simulink model "test_on_intes_cross2018_acc"  (R2018b)
settings: Solver=FixedStepAuto  StartTime=0.0  StopTime=10.0  FixedStep=0.001  RelTol=1e-3
libraries: simulink x1
settings Model: Creator=lenovo  LastModifiedBy=lenovo

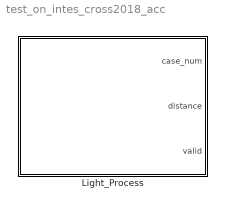
== system test_on_intes_cross2018_acc ==
  Light_Process : Subsystem

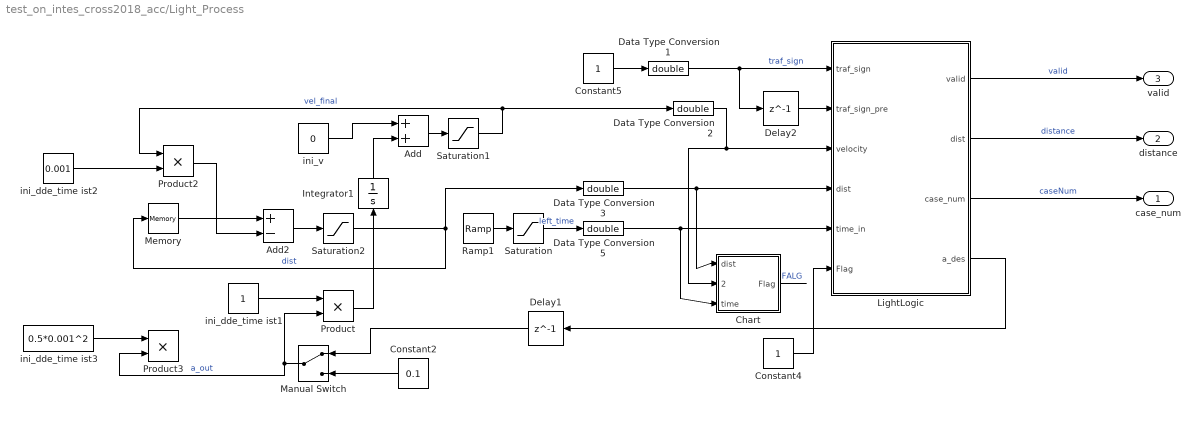
== system test_on_intes_cross2018_acc/Light_Process ==
  Add : Sum
  Add2 : Sum  Inputs=+-
  Chart : Stateflow chart  TreatAsAtomicUnit=on
  Constant2 : Constant  Value=0.1  OutDataTypeStr=single
  Constant4 : Constant  OutDataTypeStr=single
  Constant5 : Constant  OutDataTypeStr=single
  Data Type Conversion{1..3,5} (4 alike) : DataTypeConversion  OutDataTypeStr=double
  Delay1 : Delay  DelayLength=1
  Delay2 : Delay  DelayLength=1
  Integrator1 : Integrator
  LightLogic : MATLAB Function  TreatAsAtomicUnit=on
  Manual Switch : ManualSwitch
  Memory : Memory  InitialCondition=20
  Product : Product
  Product2 : Product
  Product3 : Product
  Ramp1 : simulink/Sources/Ramp  slope=-1  start=0  InitialOutput=20
  Saturation : Saturate  UpperLimit=20  LowerLimit=0
  Saturation1 : Saturate  UpperLimit=inf  LowerLimit=0
  Saturation2 : Saturate  UpperLimit=inf  LowerLimit=-10
  ini_dde_time ist1 : Constant  OutDataTypeStr=single
  ini_dde_time ist2 : Constant  Value=0.001  OutDataTypeStr=single
  ini_dde_time ist3 : Constant  Value=0.5*0.001^2  OutDataTypeStr=single
  "ini_v " : Constant  Value=0  OutDataTypeStr=single
  case_num : Outport
  distance : Outport  Port=2
  valid : Outport  Port=3
  wires:
  "ini_v "/1 -> Add/1
  Data Type Conversion1/1 -> Delay2/1, LightLogic/1(traf_sign)  "traf_sign"
  Data Type Conversion3/1 -> LightLogic/4("dist "), Chart/1(dist)
  Data Type Conversion5/1 -> LightLogic/5(time_in), Chart/3(time)
  LightLogic/3(case_num) -> case_num/1  "caseNum"
  Chart/1(Flag) -> ?  "FALG"
  Constant5/1 -> Data Type Conversion1/1
  Ramp1/1 -> Saturation/1
  Add/1 -> Saturation1/1
  Saturation/1 -> Data Type Conversion5/1  "left_time"
  Add2/1 -> Saturation2/1
  Manual Switch/1 -> Product/2, Product3/2  "a_out"
  Constant2/1 -> Manual Switch/2
  Delay1/1 -> Manual Switch/1
  Integrator1/1 -> Add/2
  ini_dde_time ist1/1 -> Product/1
  Product/1 -> Integrator1/1
  Memory/1 -> Add2/1
  ini_dde_time ist2/1 -> Product2/2
  Product2/1 -> Add2/2
  ini_dde_time ist3/1 -> Product3/1
  Constant4/1 -> LightLogic/6(Flag)
  Data Type Conversion2/1 -> Chart/2(velocity), LightLogic/3(velocity)
  Saturation1/1 -> Product2/1, Data Type Conversion2/1  "vel_final"
  Saturation2/1 -> Data Type Conversion3/1, Memory/1  "dist"
  LightLogic/1(valid) -> valid/1  "valid"
  LightLogic/2(dist) -> distance/1  "distance"
  Delay2/1 -> LightLogic/2(traf_sign_pre)
  LightLogic/4(a_des) -> Delay1/1

== stateflow chart test_on_intes_cross2018_acc/Light_Process/Chart ==
  state Off
    en:
    Flag=0;
  state init
    en:
    Flag=0;
  state On
    du:
    Flag=1;
  (default) -> Off
  On -> Off : [dist < -5 || time < 0]
  Off -> init : [time > 0 && dist > 0]
  init -> On : [time > 0 && dist > 0 && dist / (velocity + 0.0001) <= 7]
  data: dist input; velocity input; Flag output; time input

== matlab function test_on_intes_cross2018_acc/Light_Process/LightLogic ==
  data: valid output; traf_sign input; traf_sign_pre input; velocity input; dist input; time_in input; dist output; case_num output; Flag input; a_des output
function [ valid,dist,case_num,a_des] = intesec_cross( traf_sign,traf_sign_pre, velocity, dist, time_in, Flag)  
%% this is a function that provide desired velocity, and distance to traffic light;
    % input: trafic_sign with green = 0; red = 1; yellow = 2;
    %        velocity in unit of kph;
    %        dist, and time is distance(m) to cross, and traffic time left
    %        CONST_LIMIT is velocity limit at cross, which is a reference CONSTANT velocity from
    %        ACC module.
    %        v_des_pre preseve previous v_des for next step use.
    
    % output: desired velocity for ACC module, in unit of kph;
    %         dist is distance(m) to front cross;
   
    case_num = 0;
    time = time_in;
    green = 1;
    red = 3;
    yellow = 2;
    v = velocity;
%     if time == 2
%         a_des = 0;
%          v_des = 0;
%     end
    
    if (Flag == 0)
       
        a_des = 0;
        dist = 100;
        case_num = 0;
        valid = 0;
        
        return;
    end
    
    if dist < 0
        if traf_sign == green
            dist = 200;
        else
            dist = 0;
        end
    end
    
    if (Flag == 1)

        
        % CONST_LIMIT = CONST_LIMIT;
        
        ttc = dist / (v + 0.001);
        ttc = max(0,ttc);

        if traf_sign == green
            time = time + 3;
        elseif traf_sign == yellow
            traf_sign = green;
        end

        switch traf_sign
            case green
                if (ttc > time && v > 0.5 && abs(ttc) < 7)
                    valid = 1;
                    case_num = 1;
                   
                else
                    valid = 0;
                    case_num = 3;
                end

            case red
                valid = 1;
                case_num = 4;
            otherwise
                valid = 0;
                case_num = 5;
        end
        
    else
                valid = 0;
         
    end
    
    if valid == 1
        a_des = v^2 / (2 * dist);
    else 
        a_des = 1;
    end
   
end
